simulink model "q2ii"  (R2018a)
settings: Solver=FixedStepAuto  StartTime=0.0  StopTime=10.0  FixedStep=0.00001  RelTol=1e-3
libraries: simulink x1
settings Model: Creator=hp  LastModifiedBy=hp

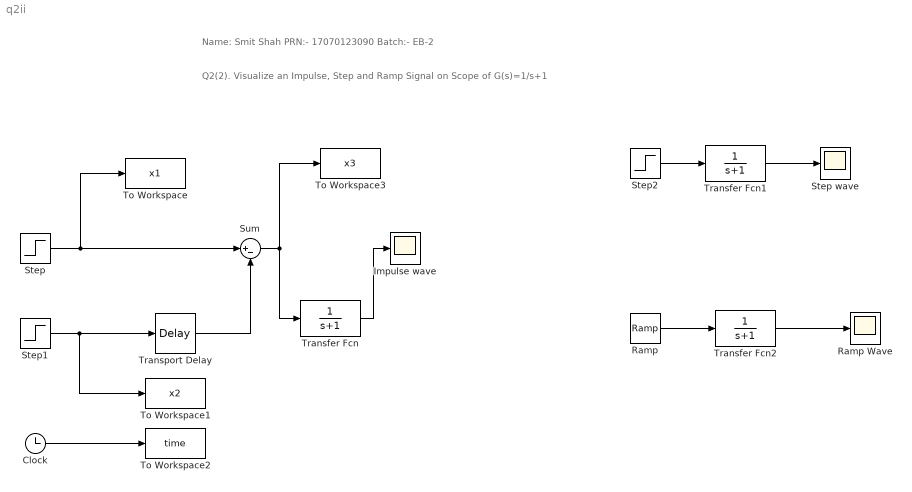
== system q2ii ==
  note: Name: Smit Shah PRN:- 17070123090 Batch:- EB-2
  note: Q2(2). Visualize an Impulse, Step and Ramp Signal on Scope of G(s)=1/s+1
  Clock : Clock
  Impulse wave : Scope
  Ramp : simulink/Sources/Ramp  slope=1  start=0  InitialOutput=0
  Ramp Wave : Scope
  Step : Step  Time=0  SampleTime=0
  Step wave : Scope
  Step1 : Step  Time=0  After=2  SampleTime=0
  Step2 : Step  Time=0  SampleTime=0
  Sum : Sum  Inputs=|+-
  To Workspace : ToWorkspace  VariableName=x1  SampleTime=-1
  To Workspace1 : ToWorkspace  VariableName=x2  SampleTime=-1
  To Workspace2 : ToWorkspace  VariableName=time  SampleTime=-1
  To Workspace3 : ToWorkspace  VariableName=x3  SampleTime=-1
  Transfer Fcn : TransferFcn  Denominator=[1 1]
  Transfer Fcn1 : TransferFcn  Denominator=[1 1]
  Transfer Fcn2 : TransferFcn  Denominator=[1 1]
  Transport Delay : TransportDelay  DelayTime=0.00001
  wires:
  Step/1 -> Sum/1, To Workspace/1
  Step1/1 -> To Workspace1/1, Transport Delay/1
  Clock/1 -> To Workspace2/1
  Transport Delay/1 -> Sum/2
  Sum/1 -> Transfer Fcn/1, To Workspace3/1
  Transfer Fcn/1 -> Impulse wave/1
  Transfer Fcn1/1 -> Step wave/1
  Step2/1 -> Transfer Fcn1/1
  Transfer Fcn2/1 -> Ramp Wave/1
  Ramp/1 -> Transfer Fcn2/1
